simulink model "Last_version_po_STO"  (R2018a)
settings: Solver=FixedStepAuto  StartTime=0.0  StopTime=inf  FixedStep=1e-3  MaxStep=1e-4  RelTol=1e-3
undefined symbols (not defined in the file): D11, Delta
libraries: powerlib x118, simulink_extras x25, powerlib_meascontrol x18, simulink x8, xpcutilitieslib x2, xpcrtudplib x2, opclib x1, sldrtlib x1
(part 2 of 3)

== system Last_version_po_STO/fourier_filter20 ==
  In1 : Inport
  Complex to Real-Imag1 : ComplexToRealImag
  Degrees to Radians : simulink_extras/Transformations/Degrees to Radians
  Fourier1 : powerlib_meascontrol/Measurements/Fourier  Freq=50  n=1  InInit=[0, 0]  Ts=0
      settings: SourceProductName=Simscape Electrical
  Gain1 : Gain  Gain=1/sqrt(2)
  Magnitude-Angle to Complex1 : MagnitudeAngleToComplex
  RMS : Outport
  Real : Outport  Port=2
  Imag : Outport  Port=3
  Complex : Outport  Port=4
  Phase : Outport  Port=5
  wires:
  Fourier1/2 -> Degrees to Radians/1
  In1/1 -> Fourier1/1
  Magnitude-Angle to Complex1/1 -> Complex/1, Complex to Real-Imag1/1
  Complex to Real-Imag1/2 -> Imag/1
  Complex to Real-Imag1/1 -> Real/1
  Degrees to Radians/1 -> Phase/1, Magnitude-Angle to Complex1/2
  Fourier1/1 -> Gain1/1
  Gain1/1 -> RMS/1, Magnitude-Angle to Complex1/1

== system Last_version_po_STO/fourier_filter21 ==
  In1 : Inport
  Complex to Real-Imag1 : ComplexToRealImag
  Degrees to Radians : simulink_extras/Transformations/Degrees to Radians
  Fourier1 : powerlib_meascontrol/Measurements/Fourier  Freq=50  n=1  InInit=[0, 0]  Ts=0
      settings: SourceProductName=Simscape Electrical
  Gain1 : Gain  Gain=1/sqrt(2)
  Magnitude-Angle to Complex1 : MagnitudeAngleToComplex
  RMS : Outport
  Real : Outport  Port=2
  Imag : Outport  Port=3
  Complex : Outport  Port=4
  Phase : Outport  Port=5
  wires:
  Gain1/1 -> Magnitude-Angle to Complex1/1, RMS/1
  Fourier1/1 -> Gain1/1
  Degrees to Radians/1 -> Magnitude-Angle to Complex1/2, Phase/1
  Complex to Real-Imag1/1 -> Real/1
  Complex to Real-Imag1/2 -> Imag/1
  Magnitude-Angle to Complex1/1 -> Complex to Real-Imag1/1, Complex/1
  In1/1 -> Fourier1/1
  Fourier1/2 -> Degrees to Radians/1

== system Last_version_po_STO/fourier_filter22 ==
  In1 : Inport
  Complex to Real-Imag1 : ComplexToRealImag
  Degrees to Radians : simulink_extras/Transformations/Degrees to Radians
  Fourier1 : powerlib_meascontrol/Measurements/Fourier  Freq=50  n=1  InInit=[0, 0]  Ts=0
      settings: SourceProductName=Simscape Electrical
  Gain1 : Gain  Gain=1/sqrt(2)
  Magnitude-Angle to Complex1 : MagnitudeAngleToComplex
  RMS : Outport
  Real : Outport  Port=2
  Imag : Outport  Port=3
  Complex : Outport  Port=4
  Phase : Outport  Port=5
  wires:
  Fourier1/2 -> Degrees to Radians/1
  In1/1 -> Fourier1/1
  Magnitude-Angle to Complex1/1 -> Complex/1, Complex to Real-Imag1/1
  Complex to Real-Imag1/2 -> Imag/1
  Complex to Real-Imag1/1 -> Real/1
  Degrees to Radians/1 -> Phase/1, Magnitude-Angle to Complex1/2
  Fourier1/1 -> Gain1/1
  Gain1/1 -> RMS/1, Magnitude-Angle to Complex1/1

== system Last_version_po_STO/fourier_filter3 ==
  In1 : Inport
  Complex to Real-Imag1 : ComplexToRealImag
  Degrees to Radians : simulink_extras/Transformations/Degrees to Radians
  Fourier1 : powerlib_meascontrol/Measurements/Fourier  Freq=50  n=1  InInit=[0, 0]  Ts=0
      settings: SourceProductName=Simscape Electrical
  Gain1 : Gain  Gain=1/sqrt(2)
  Magnitude-Angle to Complex1 : MagnitudeAngleToComplex
  RMS : Outport
  Real : Outport  Port=2
  Imag : Outport  Port=3
  Complex : Outport  Port=4
  Phase : Outport  Port=5
  wires:
  Fourier1/2 -> Degrees to Radians/1
  In1/1 -> Fourier1/1
  Magnitude-Angle to Complex1/1 -> Complex/1, Complex to Real-Imag1/1
  Complex to Real-Imag1/2 -> Imag/1
  Complex to Real-Imag1/1 -> Real/1
  Degrees to Radians/1 -> Phase/1, Magnitude-Angle to Complex1/2
  Fourier1/1 -> Gain1/1
  Gain1/1 -> RMS/1, Magnitude-Angle to Complex1/1

== system Last_version_po_STO/fourier_filter4 ==
  In1 : Inport
  Complex to Real-Imag1 : ComplexToRealImag
  Degrees to Radians : simulink_extras/Transformations/Degrees to Radians
  Fourier1 : powerlib_meascontrol/Measurements/Fourier  Freq=50  n=1  InInit=[0, 0]  Ts=0
      settings: SourceProductName=Simscape Electrical
  Gain1 : Gain  Gain=1/sqrt(2)
  Magnitude-Angle to Complex1 : MagnitudeAngleToComplex
  RMS : Outport
  Real : Outport  Port=2
  Imag : Outport  Port=3
  Complex : Outport  Port=4
  Phase : Outport  Port=5
  wires:
  Fourier1/2 -> Degrees to Radians/1
  In1/1 -> Fourier1/1
  Magnitude-Angle to Complex1/1 -> Complex/1, Complex to Real-Imag1/1
  Complex to Real-Imag1/2 -> Imag/1
  Complex to Real-Imag1/1 -> Real/1
  Degrees to Radians/1 -> Phase/1, Magnitude-Angle to Complex1/2
  Fourier1/1 -> Gain1/1
  Gain1/1 -> RMS/1, Magnitude-Angle to Complex1/1

== system Last_version_po_STO/fourier_filter5 ==
  In1 : Inport
  Complex to Real-Imag1 : ComplexToRealImag
  Degrees to Radians : simulink_extras/Transformations/Degrees to Radians
  Fourier1 : powerlib_meascontrol/Measurements/Fourier  Freq=50  n=1  InInit=[0, 0]  Ts=0
      settings: SourceProductName=Simscape Electrical
  Gain1 : Gain  Gain=1/sqrt(2)
  Magnitude-Angle to Complex1 : MagnitudeAngleToComplex
  RMS : Outport
  Real : Outport  Port=2
  Imag : Outport  Port=3
  Complex : Outport  Port=4
  Phase : Outport  Port=5
  wires:
  Fourier1/2 -> Degrees to Radians/1
  In1/1 -> Fourier1/1
  Magnitude-Angle to Complex1/1 -> Complex/1, Complex to Real-Imag1/1
  Complex to Real-Imag1/2 -> Imag/1
  Complex to Real-Imag1/1 -> Real/1
  Degrees to Radians/1 -> Phase/1, Magnitude-Angle to Complex1/2
  Fourier1/1 -> Gain1/1
  Gain1/1 -> RMS/1, Magnitude-Angle to Complex1/1

== system Last_version_po_STO/fourier_filter6 ==
  In1 : Inport
  Complex to Real-Imag1 : ComplexToRealImag
  Degrees to Radians : simulink_extras/Transformations/Degrees to Radians
  Fourier1 : powerlib_meascontrol/Measurements/Fourier  Freq=50  n=1  InInit=[0, 0]  Ts=0
      settings: SourceProductName=Simscape Electrical
  Gain1 : Gain  Gain=1/sqrt(2)
  Magnitude-Angle to Complex1 : MagnitudeAngleToComplex
  RMS : Outport
  Real : Outport  Port=2
  Imag : Outport  Port=3
  Complex : Outport  Port=4
  Phase : Outport  Port=5
  wires:
  Fourier1/2 -> Degrees to Radians/1
  In1/1 -> Fourier1/1
  Magnitude-Angle to Complex1/1 -> Complex/1, Complex to Real-Imag1/1
  Complex to Real-Imag1/2 -> Imag/1
  Complex to Real-Imag1/1 -> Real/1
  Degrees to Radians/1 -> Phase/1, Magnitude-Angle to Complex1/2
  Fourier1/1 -> Gain1/1
  Gain1/1 -> RMS/1, Magnitude-Angle to Complex1/1

== system Last_version_po_STO/fourier_filter8 ==
  In1 : Inport
  Complex to Real-Imag1 : ComplexToRealImag
  Degrees to Radians : simulink_extras/Transformations/Degrees to Radians
  Fourier1 : powerlib_meascontrol/Measurements/Fourier  Freq=50  n=1  InInit=[0, 0]  Ts=0
      settings: SourceProductName=Simscape Electrical
  Gain1 : Gain  Gain=1/sqrt(2)
  Magnitude-Angle to Complex1 : MagnitudeAngleToComplex
  RMS : Outport
  Real : Outport  Port=2
  Imag : Outport  Port=3
  Complex : Outport  Port=4
  Phase : Outport  Port=5
  wires:
  Gain1/1 -> Magnitude-Angle to Complex1/1, RMS/1
  Fourier1/1 -> Gain1/1
  Degrees to Radians/1 -> Magnitude-Angle to Complex1/2, Phase/1
  Complex to Real-Imag1/1 -> Real/1
  Complex to Real-Imag1/2 -> Imag/1
  Magnitude-Angle to Complex1/1 -> Complex to Real-Imag1/1, Complex/1
  In1/1 -> Fourier1/1
  Fourier1/2 -> Degrees to Radians/1

== system Last_version_po_STO/relay_t ==
  In : Inport
  t_vv : Inport  Port=2
  Data Type Conversion : DataTypeConversion  OutDataTypeStr=double
  Integrator1 : Integrator  ExternalReset=rising  LimitOutput=on  UpperSaturationLimit=10000
  Logical Operator2 : Logic  Operator=NOT  AllPortsSameDT=off  OutDataTypeStr=boolean
  Relational Operator : RelationalOperator  Operator=>  OutDataTypeStr=boolean  RndMeth=Nearest
  Out : Outport
  wires:
  Logical Operator2/1 -> Integrator1/2
  In/1 -> Data Type Conversion/1, Logical Operator2/1
  Relational Operator/1 -> Out/1
  Integrator1/1 -> Relational Operator/1
  t_vv/1 -> Relational Operator/2
  Data Type Conversion/1 -> Integrator1/1

== system Last_version_po_STO/KZ_simulation/relay_t ==
  In : Inport
  t_vv : Inport  Port=2
  Data Type Conversion : DataTypeConversion  OutDataTypeStr=double
  Integrator1 : Integrator  ExternalReset=rising  LimitOutput=on  UpperSaturationLimit=10000
  Logical Operator2 : Logic  Operator=NOT  AllPortsSameDT=off  OutDataTypeStr=boolean
  Relational Operator : RelationalOperator  Operator=>  OutDataTypeStr=boolean  RndMeth=Nearest
  Out : Outport
  wires:
  Logical Operator2/1 -> Integrator1/2
  In/1 -> Data Type Conversion/1, Logical Operator2/1
  Relational Operator/1 -> Out/1
  Integrator1/1 -> Relational Operator/1
  t_vv/1 -> Relational Operator/2
  Data Type Conversion/1 -> Integrator1/1

== system Last_version_po_STO/KZ_simulation/relay_t1 ==
  In : Inport
  t_vv : Inport  Port=2
  Data Type Conversion : DataTypeConversion  OutDataTypeStr=double
  Integrator1 : Integrator  ExternalReset=rising  LimitOutput=on  UpperSaturationLimit=10000
  Logical Operator2 : Logic  Operator=NOT  AllPortsSameDT=off  OutDataTypeStr=boolean
  Relational Operator : RelationalOperator  Operator=>  OutDataTypeStr=boolean  RndMeth=Nearest
  Out : Outport
  wires:
  Data Type Conversion/1 -> Integrator1/1
  t_vv/1 -> Relational Operator/2
  Integrator1/1 -> Relational Operator/1
  Relational Operator/1 -> Out/1
  In/1 -> Logical Operator2/1, Data Type Conversion/1
  Logical Operator2/1 -> Integrator1/2

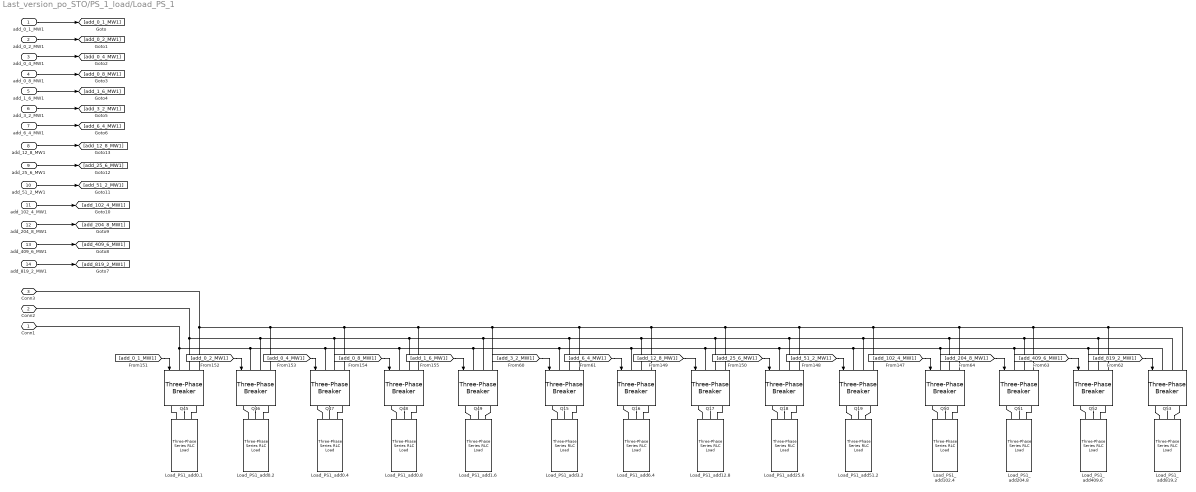
== system Last_version_po_STO/PS_1_load/Load_PS_1 ==
  add_0_1_MW1 : Inport
  add_0_2_MW1 : Inport  Port=2
  add_0_4_MW1 : Inport  Port=3
  add_0_8_MW1 : Inport  Port=4
  add_1_6_MW1 : Inport  Port=5
  add_3_2_MW1 : Inport  Port=6
  add_6_4_MW1 : Inport  Port=7
  add_12_8_MW1 : Inport  Port=8
  add_25_6_MW1 : Inport  Port=9
  add_51_2_MW1 : Inport  Port=10
  add_102_4_MW1 : Inport  Port=11
  add_204_8_MW1 : Inport  Port=12
  add_409_6_MW1 : Inport  Port=13
  add_819_2_MW1 : Inport  Port=14
  Load_PS1_add0.1 : powerlib/Elements/Three-Phase Series RLC Load  LConnTagsString=A|B|C  Configuration=Y (grounded)  NominalVoltage=330e3  Vabc=[1e3 1e3 1e3]  Vabcp=[1e3 1e3 1e3]  NominalFrequency=50  UnbalancedPower=off  ActivePower=0.1e6  InductivePower=0  CapacitivePower=0  Pabc=[10e3 9e3 11e3]  QLabc=[100 90 110]  QCabc=[100 90 110]  Pabcp=[10e3 9e3 11e3]  QLabcp=[100 90 110]  QCabcp=[100 90 110]  Measurements=None  LoadType=constant Z
      settings: SourceProductName=Simscape Electrical
  Load_PS1_add0.2 : powerlib/Elements/Three-Phase Series RLC Load  LConnTagsString=A|B|C  Configuration=Y (grounded)  NominalVoltage=330e3  Vabc=[1e3 1e3 1e3]  Vabcp=[1e3 1e3 1e3]  NominalFrequency=50  UnbalancedPower=off  ActivePower=0.2e6  InductivePower=0  CapacitivePower=0  Pabc=[10e3 9e3 11e3]  QLabc=[100 90 110]  QCabc=[100 90 110]  Pabcp=[10e3 9e3 11e3]  QLabcp=[100 90 110]  QCabcp=[100 90 110]  Measurements=None  LoadType=constant Z
      settings: SourceProductName=Simscape Electrical
  Load_PS1_add0.4 : powerlib/Elements/Three-Phase Series RLC Load  LConnTagsString=A|B|C  Configuration=Y (grounded)  NominalVoltage=330e3  Vabc=[1e3 1e3 1e3]  Vabcp=[1e3 1e3 1e3]  NominalFrequency=50  UnbalancedPower=off  ActivePower=0.4e6  InductivePower=0  CapacitivePower=0  Pabc=[10e3 9e3 11e3]  QLabc=[100 90 110]  QCabc=[100 90 110]  Pabcp=[10e3 9e3 11e3]  QLabcp=[100 90 110]  QCabcp=[100 90 110]  Measurements=None  LoadType=constant Z
      settings: SourceProductName=Simscape Electrical
  Load_PS1_add0.8 : powerlib/Elements/Three-Phase Series RLC Load  LConnTagsString=A|B|C  Configuration=Y (grounded)  NominalVoltage=330e3  Vabc=[1e3 1e3 1e3]  Vabcp=[1e3 1e3 1e3]  NominalFrequency=50  UnbalancedPower=off  ActivePower=0.8e6  InductivePower=0  CapacitivePower=0  Pabc=[10e3 9e3 11e3]  QLabc=[100 90 110]  QCabc=[100 90 110]  Pabcp=[10e3 9e3 11e3]  QLabcp=[100 90 110]  QCabcp=[100 90 110]  Measurements=None  LoadType=constant Z
      settings: SourceProductName=Simscape Electrical
  Load_PS1_add1.6 : powerlib/Elements/Three-Phase Series RLC Load  LConnTagsString=A|B|C  Configuration=Y (grounded)  NominalVoltage=330e3  Vabc=[1e3 1e3 1e3]  Vabcp=[1e3 1e3 1e3]  NominalFrequency=50  UnbalancedPower=off  ActivePower=1.6e6  InductivePower=0  CapacitivePower=0  Pabc=[10e3 9e3 11e3]  QLabc=[100 90 110]  QCabc=[100 90 110]  Pabcp=[10e3 9e3 11e3]  QLabcp=[100 90 110]  QCabcp=[100 90 110]  Measurements=None  LoadType=constant Z
      settings: SourceProductName=Simscape Electrical
  Load_PS1_add102.4 : powerlib/Elements/Three-Phase Series RLC Load  LConnTagsString=A|B|C  Configuration=Y (grounded)  NominalVoltage=330e3  Vabc=[1e3 1e3 1e3]  Vabcp=[1e3 1e3 1e3]  NominalFrequency=50  UnbalancedPower=off  ActivePower=102.4e6  InductivePower=0  CapacitivePower=0  Pabc=[10e3 9e3 11e3]  QLabc=[100 90 110]  QCabc=[100 90 110]  Pabcp=[10e3 9e3 11e3]  QLabcp=[100 90 110]  QCabcp=[100 90 110]  Measurements=None  LoadType=constant Z
      settings: SourceProductName=Simscape Electrical
  Load_PS1_add12.8 : powerlib/Elements/Three-Phase Series RLC Load  LConnTagsString=A|B|C  Configuration=Y (grounded)  NominalVoltage=330e3  Vabc=[1e3 1e3 1e3]  Vabcp=[1e3 1e3 1e3]  NominalFrequency=50  UnbalancedPower=off  ActivePower=12.8e6  InductivePower=0  CapacitivePower=0  Pabc=[10e3 9e3 11e3]  QLabc=[100 90 110]  QCabc=[100 90 110]  Pabcp=[10e3 9e3 11e3]  QLabcp=[100 90 110]  QCabcp=[100 90 110]  Measurements=None  LoadType=constant Z
      settings: SourceProductName=Simscape Electrical
  Load_PS1_add204.8 : powerlib/Elements/Three-Phase Series RLC Load  LConnTagsString=A|B|C  Configuration=Y (grounded)  NominalVoltage=330e3  Vabc=[1e3 1e3 1e3]  Vabcp=[1e3 1e3 1e3]  NominalFrequency=50  UnbalancedPower=off  ActivePower=204.8e6  InductivePower=0  CapacitivePower=0  Pabc=[10e3 9e3 11e3]  QLabc=[100 90 110]  QCabc=[100 90 110]  Pabcp=[10e3 9e3 11e3]  QLabcp=[100 90 110]  QCabcp=[100 90 110]  Measurements=None  LoadType=constant Z
      settings: SourceProductName=Simscape Electrical
  Load_PS1_add25.6 : powerlib/Elements/Three-Phase Series RLC Load  LConnTagsString=A|B|C  Configuration=Y (grounded)  NominalVoltage=330e3  Vabc=[1e3 1e3 1e3]  Vabcp=[1e3 1e3 1e3]  NominalFrequency=50  UnbalancedPower=off  ActivePower=25.6e6  InductivePower=0  CapacitivePower=0  Pabc=[10e3 9e3 11e3]  QLabc=[100 90 110]  QCabc=[100 90 110]  Pabcp=[10e3 9e3 11e3]  QLabcp=[100 90 110]  QCabcp=[100 90 110]  Measurements=None  LoadType=constant Z
      settings: SourceProductName=Simscape Electrical
  Load_PS1_add3.2 : powerlib/Elements/Three-Phase Series RLC Load  LConnTagsString=A|B|C  Configuration=Y (grounded)  NominalVoltage=330e3  Vabc=[1e3 1e3 1e3]  Vabcp=[1e3 1e3 1e3]  NominalFrequency=50  UnbalancedPower=off  ActivePower=3.2e6  InductivePower=0  CapacitivePower=0  Pabc=[10e3 9e3 11e3]  QLabc=[100 90 110]  QCabc=[100 90 110]  Pabcp=[10e3 9e3 11e3]  QLabcp=[100 90 110]  QCabcp=[100 90 110]  Measurements=None  LoadType=constant Z
      settings: SourceProductName=Simscape Electrical
  Load_PS1_add409.6 : powerlib/Elements/Three-Phase Series RLC Load  LConnTagsString=A|B|C  Configuration=Y (grounded)  NominalVoltage=330e3  Vabc=[1e3 1e3 1e3]  Vabcp=[1e3 1e3 1e3]  NominalFrequency=50  UnbalancedPower=off  ActivePower=409.6e6  InductivePower=0  CapacitivePower=0  Pabc=[10e3 9e3 11e3]  QLabc=[100 90 110]  QCabc=[100 90 110]  Pabcp=[10e3 9e3 11e3]  QLabcp=[100 90 110]  QCabcp=[100 90 110]  Measurements=None  LoadType=constant Z
      settings: SourceProductName=Simscape Electrical
  Load_PS1_add51.2 : powerlib/Elements/Three-Phase Series RLC Load  LConnTagsString=A|B|C  Configuration=Y (grounded)  NominalVoltage=330e3  Vabc=[1e3 1e3 1e3]  Vabcp=[1e3 1e3 1e3]  NominalFrequency=50  UnbalancedPower=off  ActivePower=51.2e6  InductivePower=0  CapacitivePower=0  Pabc=[10e3 9e3 11e3]  QLabc=[100 90 110]  QCabc=[100 90 110]  Pabcp=[10e3 9e3 11e3]  QLabcp=[100 90 110]  QCabcp=[100 90 110]  Measurements=None  LoadType=constant Z
      settings: SourceProductName=Simscape Electrical
  Load_PS1_add6.4 : powerlib/Elements/Three-Phase Series RLC Load  LConnTagsString=A|B|C  Configuration=Y (grounded)  NominalVoltage=330e3  Vabc=[1e3 1e3 1e3]  Vabcp=[1e3 1e3 1e3]  NominalFrequency=50  UnbalancedPower=off  ActivePower=6.4e6  InductivePower=0  CapacitivePower=0  Pabc=[10e3 9e3 11e3]  QLabc=[100 90 110]  QCabc=[100 90 110]  Pabcp=[10e3 9e3 11e3]  QLabcp=[100 90 110]  QCabcp=[100 90 110]  Measurements=None  LoadType=constant Z
      settings: SourceProductName=Simscape Electrical
  Load_PS1_add819.2 : powerlib/Elements/Three-Phase Series RLC Load  LConnTagsString=A|B|C  Configuration=Y (grounded)  NominalVoltage=330e3  Vabc=[1e3 1e3 1e3]  Vabcp=[1e3 1e3 1e3]  NominalFrequency=50  UnbalancedPower=off  ActivePower=819.2e6  InductivePower=0  CapacitivePower=0  Pabc=[10e3 9e3 11e3]  QLabc=[100 90 110]  QCabc=[100 90 110]  Pabcp=[10e3 9e3 11e3]  QLabcp=[100 90 110]  QCabcp=[100 90 110]  Measurements=None  LoadType=constant Z
      settings: SourceProductName=Simscape Electrical
  Q{15..19,45..53} (14 alike) : powerlib/Elements/Three-Phase Breaker  InitialState=open  SwitchA=on  SwitchB=on  SwitchC=on  SwitchTimes="[1/60  5/60]"  External=on  BreakerResistance=0.01  SnubberResistance=1e6  SnubberCapacitance=inf  Measurements=None
      settings: SourceProductName=Simscape Electrical
  Conn1 : PMIOPort  Side=Left
  Conn2 : PMIOPort  Port=2  Side=Left
  Conn3 : PMIOPort  Port=3  Side=Left
  wires:
  [add_0_8_MW1] -> Q48/1
  [add_1_6_MW1] -> Q49/1
  [add_6_4_MW1] -> Q16/1
  [add_3_2_MW1] -> Q15/1
  [add_204_8_MW1] -> Q51/1
  [add_25_6_MW1] -> Q18/1
  [add_0_4_MW1] -> Q47/1
  [add_0_1_MW1] -> Q45/1
  [add_0_2_MW1] -> Q46/1
  [add_409_6_MW1] -> Q52/1
  [add_51_2_MW1] -> Q19/1
  [add_819_2_MW1] -> Q53/1
  [add_12_8_MW1] -> Q17/1
  [add_102_4_MW1] -> Q50/1
  add_0_1_MW1/1 -> [add_0_1_MW1]
  add_0_2_MW1/1 -> [add_0_2_MW1]
  add_0_4_MW1/1 -> [add_0_4_MW1]
  add_0_8_MW1/1 -> [add_0_8_MW1]
  add_1_6_MW1/1 -> [add_1_6_MW1]
  add_3_2_MW1/1 -> [add_3_2_MW1]
  add_6_4_MW1/1 -> [add_6_4_MW1]
  add_25_6_MW1/1 -> [add_25_6_MW1]
  add_51_2_MW1/1 -> [add_51_2_MW1]
  add_102_4_MW1/1 -> [add_102_4_MW1]
  add_204_8_MW1/1 -> [add_204_8_MW1]
  add_409_6_MW1/1 -> [add_409_6_MW1]
  add_819_2_MW1/1 -> [add_819_2_MW1]
  add_12_8_MW1/1 -> [add_12_8_MW1]
  connections:
  Q52/LConn1 -- Q48/LConn1 -- Q47/LConn1 -- Q46/LConn1 -- Conn1/RConn1 -- Q45/LConn1 -- Q49/LConn1 -- Q15/LConn1 -- Q16/LConn1 -- Q17/LConn1 -- Q18/LConn1 -- Q19/LConn1 -- Q50/LConn1 -- Q51/LConn1 -- Q53/LConn1
  Load_PS1_add12.8/LConn2 -- Q17/RConn2
  Q52/LConn3 -- Q48/LConn3 -- Q47/LConn3 -- Q46/LConn3 -- Conn3/RConn1 -- Q45/LConn3 -- Q49/LConn3 -- Q15/LConn3 -- Q16/LConn3 -- Q17/LConn3 -- Q18/LConn3 -- Q19/LConn3 -- Q50/LConn3 -- Q51/LConn3 -- Q53/LConn3
  Q52/LConn2 -- Q48/LConn2 -- Q47/LConn2 -- Q46/LConn2 -- Conn2/RConn1 -- Q45/LConn2 -- Q49/LConn2 -- Q15/LConn2 -- Q16/LConn2 -- Q17/LConn2 -- Q18/LConn2 -- Q19/LConn2 -- Q50/LConn2 -- Q51/LConn2 -- Q53/LConn2
  Q49/RConn1 -- Load_PS1_add1.6/LConn1
  Load_PS1_add6.4/LConn1 -- Q16/RConn1
  Q53/RConn1 -- Load_PS1_add819.2/LConn1
  Load_PS1_add1.6/LConn2 -- Q49/RConn2
  Load_PS1_add409.6/LConn3 -- Q52/RConn3
  Load_PS1_add0.2/LConn1 -- Q46/RConn1
  Load_PS1_add102.4/LConn3 -- Q50/RConn3
  Q45/RConn2 -- Load_PS1_add0.1/LConn2
  Load_PS1_add0.1/LConn3 -- Q45/RConn3
  Load_PS1_add0.4/LConn1 -- Q47/RConn1
  Q48/RConn2 -- Load_PS1_add0.8/LConn2
  Q49/RConn3 -- Load_PS1_add1.6/LConn3
  Load_PS1_add0.8/LConn3 -- Q48/RConn3
  Q16/RConn2 -- Load_PS1_add6.4/LConn2
  Q19/RConn3 -- Load_PS1_add51.2/LConn3
  Load_PS1_add0.8/LConn1 -- Q48/RConn1
  Q53/RConn3 -- Load_PS1_add819.2/LConn3
  Q19/RConn1 -- Load_PS1_add51.2/LConn1
  Load_PS1_add25.6/LConn1 -- Q18/RConn1
  Load_PS1_add25.6/LConn3 -- Q18/RConn3
  Load_PS1_add0.4/LConn2 -- Q47/RConn2
  Load_PS1_add12.8/LConn1 -- Q17/RConn1
  Load_PS1_add102.4/LConn1 -- Q50/RConn1
  Load_PS1_add819.2/LConn2 -- Q53/RConn2
  Load_PS1_add0.1/LConn1 -- Q45/RConn1
  Q52/RConn2 -- Load_PS1_add409.6/LConn2
  Q18/RConn2 -- Load_PS1_add25.6/LConn2
  Load_PS1_add0.4/LConn3 -- Q47/RConn3
  Load_PS1_add6.4/LConn3 -- Q16/RConn3
  Q46/RConn2 -- Load_PS1_add0.2/LConn2
  Load_PS1_add409.6/LConn1 -- Q52/RConn1
  Load_PS1_add51.2/LConn2 -- Q19/RConn2
  Load_PS1_add3.2/LConn3 -- Q15/RConn3
  Load_PS1_add0.2/LConn3 -- Q46/RConn3
  Load_PS1_add204.8/LConn3 -- Q51/RConn3
  Load_PS1_add3.2/LConn1 -- Q15/RConn1
  Load_PS1_add204.8/LConn2 -- Q51/RConn2
  Load_PS1_add12.8/LConn3 -- Q17/RConn3
  Q50/RConn2 -- Load_PS1_add102.4/LConn2
  Load_PS1_add204.8/LConn1 -- Q51/RConn1
  Load_PS1_add3.2/LConn2 -- Q15/RConn2

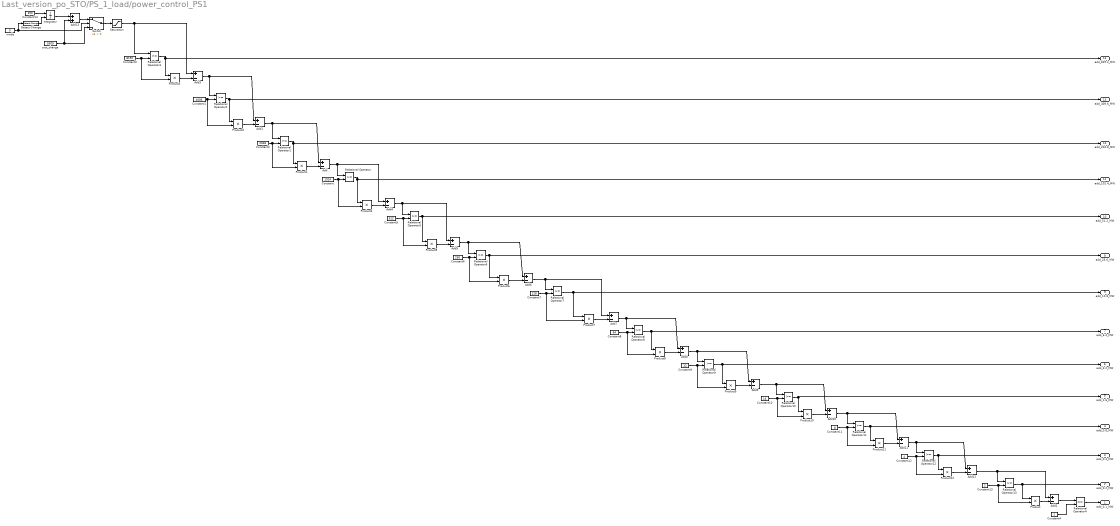
== system Last_version_po_STO/PS_1_load/power_control_PS1 ==
  Add{,1..12} (13 alike) : Sum  Inputs=+-
  Add13 : Sum
  Constant : Constant  Value=1024
  Constant1 : Constant  Value=4096
  Constant10 : Constant  Value=16
  Constant11 : Constant  Value=8
  Constant12 : Constant  Value=4
  Constant13 : Constant  Value=2
  Constant14 : Constant  Value=350
  Constant2 : Constant  Value=2048
  Constant3 : Constant  Value=8192
  Constant4 : Constant
  Constant5 : Constant  Value=512
  Constant6 : Constant  Value=256
  Constant7 : Constant  Value=128
  Constant8 : Constant  Value=64
  Constant9 : Constant  Value=32
  Detect Change : simulink/Logic and Bit Operations/Detect Change  vinit=0  OutDataTypeStr=boolean
  Integrator : Integrator  ExternalReset=rising
  Product{,1..12} (13 alike) : Product
  Relational Operator{,1..3,5..13} (13 alike) : RelationalOperator  OutDataTypeStr=boolean  RndMeth=Simplest
  Relational Operator4 : RelationalOperator  Operator===  OutDataTypeStr=boolean  RndMeth=Simplest
  Saturation : Saturate  UpperLimit=10000  LowerLimit=0
  Switch : Switch  Criteria=u2 > Threshold
  cnst_change : Constant  Value=5509
  mode : Constant  Value=0
  add_0.1_MW : Outport
  add_0.2_MW : Outport  Port=2
  add_0.4_MW : Outport  Port=3
  add_0.8_MW : Outport  Port=4
  add_1.6_MW : Outport  Port=5
  add_3.2_MW : Outport  Port=6
  add_6.4_MW : Outport  Port=7
  add_12.8_MW : Outport  Port=8
  add_25.6_MW : Outport  Port=9
  add_51.2_MW : Outport  Port=10
  add_102.4_MW : Outport  Port=11
  add_204.8_MW : Outport  Port=12
  add_409.6_MW : Outport  Port=13
  add_819.2_MW : Outport  Port=14
  wires:
  Constant3/1 -> Relational Operator3/2, Product3/2
  Add2/1 -> Relational Operator4/1
  Relational Operator2/1 -> Product2/1, add_409.6_MW/1
  Add1/1 -> Relational Operator1/1, Add/1
  Constant1/1 -> Relational Operator2/2, Product2/2
  Product2/1 -> Add1/2
  Relational Operator4/1 -> add_0.1_MW/1
  Constant4/1 -> Relational Operator4/2
  Product1/1 -> Add/2
  Product/1 -> Add2/2
  Add/1 -> Add4/1, Relational Operator/1
  Relational Operator/1 -> add_102.4_MW/1, Product4/1
  Constant2/1 -> Relational Operator1/2, Product1/2
  Relational Operator1/1 -> Product1/1, add_204.8_MW/1
  Constant/1 -> Product4/2, Relational Operator/2
  Product3/1 -> Add3/2
  Add3/1 -> Relational Operator2/1, Add1/1
  Relational Operator3/1 -> Product3/1, add_819.2_MW/1
  Constant5/1 -> Product5/2, Relational Operator5/2
  Add4/1 -> Add5/1, Relational Operator5/1
  Product4/1 -> Add4/2
  Product5/1 -> Add5/2
  Add5/1 -> Relational Operator6/1, Add6/1
  Constant6/1 -> Product6/2, Relational Operator6/2
  Constant7/1 -> Product7/2, Relational Operator7/2
  Add6/1 -> Add7/1, Relational Operator7/1
  Product6/1 -> Add6/2
  Relational Operator5/1 -> Product5/1, add_51.2_MW/1
  Relational Operator6/1 -> add_25.6_MW/1, Product6/1
  Product7/1 -> Add7/2
  Add7/1 -> Add8/1, Relational Operator8/1
  Constant8/1 -> Product8/2, Relational Operator8/2
  Constant9/1 -> Product9/2, Relational Operator9/2
  Add8/1 -> Add9/1, Relational Operator9/1
  Product8/1 -> Add8/2
  Product9/1 -> Add9/2
  Add9/1 -> Add10/1, Relational Operator10/1
  Constant10/1 -> Product10/2, Relational Operator10/2
  Constant11/1 -> Product11/2, Relational Operator11/2
  Add10/1 -> Add11/1, Relational Operator11/1
  Product10/1 -> Add10/2
  Product11/1 -> Add11/2
  Add11/1 -> Add12/1, Relational Operator12/1
  Constant12/1 -> Product12/2, Relational Operator12/2
  Constant13/1 -> Product/2, Relational Operator13/2
  Add12/1 -> Add2/1, Relational Operator13/1
  Product12/1 -> Add12/2
  Relational Operator7/1 -> add_12.8_MW/1, Product7/1
  Relational Operator8/1 -> add_6.4_MW/1, Product8/1
  Relational Operator9/1 -> add_3.2_MW/1, Product9/1
  Relational Operator10/1 -> add_1.6_MW/1, Product10/1
  Relational Operator11/1 -> add_0.8_MW/1, Product11/1
  Relational Operator12/1 -> add_0.4_MW/1, Product12/1
  Relational Operator13/1 -> add_0.2_MW/1, Product/1
  Constant14/1 -> Integrator/1
  cnst_change/1 -> Switch/3, Add13/2
  Saturation/1 -> Relational Operator3/1, Add3/1
  Switch/1 -> Saturation/1
  Add13/1 -> Switch/1
  Integrator/1 -> Add13/1
  mode/1 -> Detect Change/1, Switch/2
  Detect Change/1 -> Integrator/2

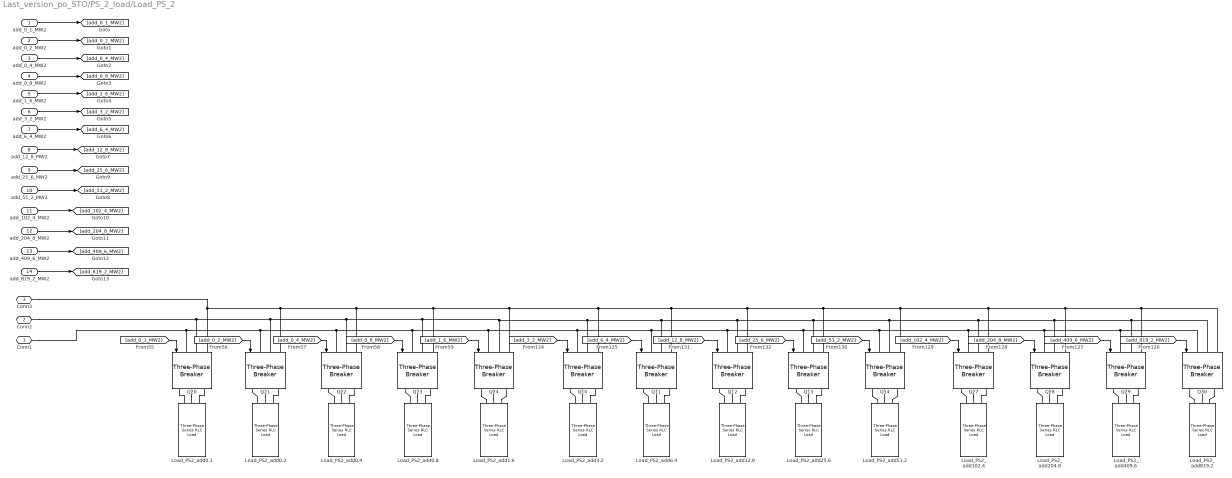
== system Last_version_po_STO/PS_2_load/Load_PS_2 ==
  add_0_1_MW2 : Inport
  add_0_2_MW2 : Inport  Port=2
  add_0_4_MW2 : Inport  Port=3
  add_0_8_MW2 : Inport  Port=4
  add_1_6_MW2 : Inport  Port=5
  add_3_2_MW2 : Inport  Port=6
  add_6_4_MW2 : Inport  Port=7
  add_12_8_MW2 : Inport  Port=8
  add_25_6_MW2 : Inport  Port=9
  add_51_2_MW2 : Inport  Port=10
  add_102_4_MW2 : Inport  Port=11
  add_204_8_MW2 : Inport  Port=12
  add_409_6_MW2 : Inport  Port=13
  add_819_2_MW2 : Inport  Port=14
  Load_PS2_add0.1 : powerlib/Elements/Three-Phase Series RLC Load  LConnTagsString=A|B|C  Configuration=Y (grounded)  NominalVoltage=330e3  Vabc=[1e3 1e3 1e3]  Vabcp=[1e3 1e3 1e3]  NominalFrequency=50  UnbalancedPower=off  ActivePower=0.1e6  InductivePower=0  CapacitivePower=0  Pabc=[10e3 9e3 11e3]  QLabc=[100 90 110]  QCabc=[100 90 110]  Pabcp=[10e3 9e3 11e3]  QLabcp=[100 90 110]  QCabcp=[100 90 110]  Measurements=None  LoadType=constant Z
      settings: SourceProductName=Simscape Electrical
  Load_PS2_add0.2 : powerlib/Elements/Three-Phase Series RLC Load  LConnTagsString=A|B|C  Configuration=Y (grounded)  NominalVoltage=330e3  Vabc=[1e3 1e3 1e3]  Vabcp=[1e3 1e3 1e3]  NominalFrequency=50  UnbalancedPower=off  ActivePower=0.2e6  InductivePower=0  CapacitivePower=0  Pabc=[10e3 9e3 11e3]  QLabc=[100 90 110]  QCabc=[100 90 110]  Pabcp=[10e3 9e3 11e3]  QLabcp=[100 90 110]  QCabcp=[100 90 110]  Measurements=None  LoadType=constant Z
      settings: SourceProductName=Simscape Electrical
  Load_PS2_add0.4 : powerlib/Elements/Three-Phase Series RLC Load  LConnTagsString=A|B|C  Configuration=Y (grounded)  NominalVoltage=330e3  Vabc=[1e3 1e3 1e3]  Vabcp=[1e3 1e3 1e3]  NominalFrequency=50  UnbalancedPower=off  ActivePower=0.4e6  InductivePower=0  CapacitivePower=0  Pabc=[10e3 9e3 11e3]  QLabc=[100 90 110]  QCabc=[100 90 110]  Pabcp=[10e3 9e3 11e3]  QLabcp=[100 90 110]  QCabcp=[100 90 110]  Measurements=None  LoadType=constant Z
      settings: SourceProductName=Simscape Electrical
  Load_PS2_add0.8 : powerlib/Elements/Three-Phase Series RLC Load  LConnTagsString=A|B|C  Configuration=Y (grounded)  NominalVoltage=330e3  Vabc=[1e3 1e3 1e3]  Vabcp=[1e3 1e3 1e3]  NominalFrequency=50  UnbalancedPower=off  ActivePower=0.8e6  InductivePower=0  CapacitivePower=0  Pabc=[10e3 9e3 11e3]  QLabc=[100 90 110]  QCabc=[100 90 110]  Pabcp=[10e3 9e3 11e3]  QLabcp=[100 90 110]  QCabcp=[100 90 110]  Measurements=None  LoadType=constant Z
      settings: SourceProductName=Simscape Electrical
  Load_PS2_add1.6 : powerlib/Elements/Three-Phase Series RLC Load  LConnTagsString=A|B|C  Configuration=Y (grounded)  NominalVoltage=330e3  Vabc=[1e3 1e3 1e3]  Vabcp=[1e3 1e3 1e3]  NominalFrequency=50  UnbalancedPower=off  ActivePower=1.6e6  InductivePower=0  CapacitivePower=0  Pabc=[10e3 9e3 11e3]  QLabc=[100 90 110]  QCabc=[100 90 110]  Pabcp=[10e3 9e3 11e3]  QLabcp=[100 90 110]  QCabcp=[100 90 110]  Measurements=None  LoadType=constant Z
      settings: SourceProductName=Simscape Electrical
  Load_PS2_add102.4 : powerlib/Elements/Three-Phase Series RLC Load  LConnTagsString=A|B|C  Configuration=Y (grounded)  NominalVoltage=330e3  Vabc=[1e3 1e3 1e3]  Vabcp=[1e3 1e3 1e3]  NominalFrequency=50  UnbalancedPower=off  ActivePower=102.4e6  InductivePower=0  CapacitivePower=0  Pabc=[10e3 9e3 11e3]  QLabc=[100 90 110]  QCabc=[100 90 110]  Pabcp=[10e3 9e3 11e3]  QLabcp=[100 90 110]  QCabcp=[100 90 110]  Measurements=None  LoadType=constant Z
      settings: SourceProductName=Simscape Electrical
  Load_PS2_add12.8 : powerlib/Elements/Three-Phase Series RLC Load  LConnTagsString=A|B|C  Configuration=Y (grounded)  NominalVoltage=330e3  Vabc=[1e3 1e3 1e3]  Vabcp=[1e3 1e3 1e3]  NominalFrequency=50  UnbalancedPower=off  ActivePower=12.8e6  InductivePower=0  CapacitivePower=0  Pabc=[10e3 9e3 11e3]  QLabc=[100 90 110]  QCabc=[100 90 110]  Pabcp=[10e3 9e3 11e3]  QLabcp=[100 90 110]  QCabcp=[100 90 110]  Measurements=None  LoadType=constant Z
      settings: SourceProductName=Simscape Electrical
  Load_PS2_add204.8 : powerlib/Elements/Three-Phase Series RLC Load  LConnTagsString=A|B|C  Configuration=Y (grounded)  NominalVoltage=330e3  Vabc=[1e3 1e3 1e3]  Vabcp=[1e3 1e3 1e3]  NominalFrequency=50  UnbalancedPower=off  ActivePower=204.8e6  InductivePower=0  CapacitivePower=0  Pabc=[10e3 9e3 11e3]  QLabc=[100 90 110]  QCabc=[100 90 110]  Pabcp=[10e3 9e3 11e3]  QLabcp=[100 90 110]  QCabcp=[100 90 110]  Measurements=None  LoadType=constant Z
      settings: SourceProductName=Simscape Electrical
  Load_PS2_add25.6 : powerlib/Elements/Three-Phase Series RLC Load  LConnTagsString=A|B|C  Configuration=Y (grounded)  NominalVoltage=330e3  Vabc=[1e3 1e3 1e3]  Vabcp=[1e3 1e3 1e3]  NominalFrequency=50  UnbalancedPower=off  ActivePower=25.6e6  InductivePower=0  CapacitivePower=0  Pabc=[10e3 9e3 11e3]  QLabc=[100 90 110]  QCabc=[100 90 110]  Pabcp=[10e3 9e3 11e3]  QLabcp=[100 90 110]  QCabcp=[100 90 110]  Measurements=None  LoadType=constant Z
      settings: SourceProductName=Simscape Electrical
  Load_PS2_add3.2 : powerlib/Elements/Three-Phase Series RLC Load  LConnTagsString=A|B|C  Configuration=Y (grounded)  NominalVoltage=330e3  Vabc=[1e3 1e3 1e3]  Vabcp=[1e3 1e3 1e3]  NominalFrequency=50  UnbalancedPower=off  ActivePower=3.2e6  InductivePower=0  CapacitivePower=0  Pabc=[10e3 9e3 11e3]  QLabc=[100 90 110]  QCabc=[100 90 110]  Pabcp=[10e3 9e3 11e3]  QLabcp=[100 90 110]  QCabcp=[100 90 110]  Measurements=None  LoadType=constant Z
      settings: SourceProductName=Simscape Electrical
  Load_PS2_add409.6 : powerlib/Elements/Three-Phase Series RLC Load  LConnTagsString=A|B|C  Configuration=Y (grounded)  NominalVoltage=330e3  Vabc=[1e3 1e3 1e3]  Vabcp=[1e3 1e3 1e3]  NominalFrequency=50  UnbalancedPower=off  ActivePower=409.6e6  InductivePower=0  CapacitivePower=0  Pabc=[10e3 9e3 11e3]  QLabc=[100 90 110]  QCabc=[100 90 110]  Pabcp=[10e3 9e3 11e3]  QLabcp=[100 90 110]  QCabcp=[100 90 110]  Measurements=None  LoadType=constant Z
      settings: SourceProductName=Simscape Electrical
  Load_PS2_add51.2 : powerlib/Elements/Three-Phase Series RLC Load  LConnTagsString=A|B|C  Configuration=Y (grounded)  NominalVoltage=330e3  Vabc=[1e3 1e3 1e3]  Vabcp=[1e3 1e3 1e3]  NominalFrequency=50  UnbalancedPower=off  ActivePower=51.2e6  InductivePower=0  CapacitivePower=0  Pabc=[10e3 9e3 11e3]  QLabc=[100 90 110]  QCabc=[100 90 110]  Pabcp=[10e3 9e3 11e3]  QLabcp=[100 90 110]  QCabcp=[100 90 110]  Measurements=None  LoadType=constant Z
      settings: SourceProductName=Simscape Electrical
  Load_PS2_add6.4 : powerlib/Elements/Three-Phase Series RLC Load  LConnTagsString=A|B|C  Configuration=Y (grounded)  NominalVoltage=330e3  Vabc=[1e3 1e3 1e3]  Vabcp=[1e3 1e3 1e3]  NominalFrequency=50  UnbalancedPower=off  ActivePower=6.4e6  InductivePower=0  CapacitivePower=0  Pabc=[10e3 9e3 11e3]  QLabc=[100 90 110]  QCabc=[100 90 110]  Pabcp=[10e3 9e3 11e3]  QLabcp=[100 90 110]  QCabcp=[100 90 110]  Measurements=None  LoadType=constant Z
      settings: SourceProductName=Simscape Electrical
  Load_PS2_add819.2 : powerlib/Elements/Three-Phase Series RLC Load  LConnTagsString=A|B|C  Configuration=Y (grounded)  NominalVoltage=330e3  Vabc=[1e3 1e3 1e3]  Vabcp=[1e3 1e3 1e3]  NominalFrequency=50  UnbalancedPower=off  ActivePower=819.2e6  InductivePower=0  CapacitivePower=0  Pabc=[10e3 9e3 11e3]  QLabc=[100 90 110]  QCabc=[100 90 110]  Pabcp=[10e3 9e3 11e3]  QLabcp=[100 90 110]  QCabcp=[100 90 110]  Measurements=None  LoadType=constant Z
      settings: SourceProductName=Simscape Electrical
  Q{10..14,20..24,27..30} (14 alike) : powerlib/Elements/Three-Phase Breaker  InitialState=open  SwitchA=on  SwitchB=on  SwitchC=on  SwitchTimes="[1/60  5/60]"  External=on  BreakerResistance=0.01  SnubberResistance=1e6  SnubberCapacitance=inf  Measurements=None
      settings: SourceProductName=Simscape Electrical
  Conn1 : PMIOPort  Side=Left
  Conn2 : PMIOPort  Port=2  Side=Left
  Conn3 : PMIOPort  Port=3  Side=Left
  wires:
  [add_0_8_MW2] -> Q23/1
  [add_204_8_MW2] -> Q28/1
  [add_25_6_MW2] -> Q13/1
  [add_1_6_MW2] -> Q24/1
  [add_0_4_MW2] -> Q22/1
  [add_0_2_MW2] -> Q21/1
  [add_819_2_MW2] -> Q30/1
  [add_6_4_MW2] -> Q11/1
  [add_409_6_MW2] -> Q29/1
  [add_51_2_MW2] -> Q14/1
  [add_0_1_MW2] -> Q20/1
  [add_102_4_MW2] -> Q27/1
  [add_3_2_MW2] -> Q10/1
  [add_12_8_MW2] -> Q12/1
  add_0_1_MW2/1 -> [add_0_1_MW2]
  add_0_4_MW2/1 -> [add_0_4_MW2]
  add_0_2_MW2/1 -> [add_0_2_MW2]
  add_0_8_MW2/1 -> [add_0_8_MW2]
  add_1_6_MW2/1 -> [add_1_6_MW2]
  add_3_2_MW2/1 -> [add_3_2_MW2]
  add_6_4_MW2/1 -> [add_6_4_MW2]
  add_12_8_MW2/1 -> [add_12_8_MW2]
  add_25_6_MW2/1 -> [add_25_6_MW2]
  add_51_2_MW2/1 -> [add_51_2_MW2]
  add_102_4_MW2/1 -> [add_102_4_MW2]
  add_204_8_MW2/1 -> [add_204_8_MW2]
  add_409_6_MW2/1 -> [add_409_6_MW2]
  add_819_2_MW2/1 -> [add_819_2_MW2]
  connections:
  Load_PS2_add204.8/LConn2 -- Q28/RConn2
  Q11/RConn2 -- Load_PS2_add6.4/LConn2
  Q24/LConn3 -- Q29/LConn3 -- Q30/LConn3 -- Q28/LConn3 -- Q27/LConn3 -- Q14/LConn3 -- Q13/LConn3 -- Q12/LConn3 -- Q11/LConn3 -- Q10/LConn3 -- Q23/LConn3 -- Q22/LConn3 -- Q21/LConn3 -- Conn3/RConn1 -- Q20/LConn3
  Q24/LConn2 -- Q29/LConn2 -- Q30/LConn2 -- Q28/LConn2 -- Q27/LConn2 -- Q14/LConn2 -- Q13/LConn2 -- Q12/LConn2 -- Q11/LConn2 -- Q10/LConn2 -- Q23/LConn2 -- Q22/LConn2 -- Q21/LConn2 -- Conn2/RConn1 -- Q20/LConn2
  Load_PS2_add204.8/LConn3 -- Q28/RConn3
  Load_PS2_add0.1/LConn1 -- Q20/RConn1
  Q23/LConn1 -- Q29/LConn1 -- Q30/LConn1 -- Q28/LConn1 -- Q27/LConn1 -- Q14/LConn1 -- Q13/LConn1 -- Q12/LConn1 -- Q11/LConn1 -- Q10/LConn1 -- Q24/LConn1 -- Q22/LConn1 -- Q21/LConn1 -- Conn1/RConn1 -- Q20/LConn1
  Load_PS2_add25.6/LConn1 -- Q13/RConn1
  Load_PS2_add0.1/LConn3 -- Q20/RConn3
  Load_PS2_add0.8/LConn3 -- Q23/RConn3
  Q27/RConn2 -- Load_PS2_add102.4/LConn2
  Q30/RConn1 -- Load_PS2_add819.2/LConn1
  Load_PS2_add0.2/LConn3 -- Q21/RConn3
  Load_PS2_add1.6/LConn2 -- Q24/RConn2
  Q20/RConn2 -- Load_PS2_add0.1/LConn2
  Q24/RConn1 -- Load_PS2_add1.6/LConn1
  Load_PS2_add0.8/LConn1 -- Q23/RConn1
  Load_PS2_add0.4/LConn2 -- Q22/RConn2
  Q24/RConn3 -- Load_PS2_add1.6/LConn3
  Q29/RConn2 -- Load_PS2_add409.6/LConn2
  Q21/RConn2 -- Load_PS2_add0.2/LConn2
  Load_PS2_add3.2/LConn2 -- Q10/RConn2
  Q14/RConn1 -- Load_PS2_add51.2/LConn1
  Load_PS2_add25.6/LConn3 -- Q13/RConn3
  Load_PS2_add12.8/LConn3 -- Q12/RConn3
  Load_PS2_add12.8/LConn2 -- Q12/RConn2
  Load_PS2_add6.4/LConn3 -- Q11/RConn3
  Q14/RConn3 -- Load_PS2_add51.2/LConn3
  Q30/RConn3 -- Load_PS2_add819.2/LConn3
  Load_PS2_add102.4/LConn1 -- Q27/RConn1
  Load_PS2_add204.8/LConn1 -- Q28/RConn1
  Load_PS2_add6.4/LConn1 -- Q11/RConn1
  Load_PS2_add409.6/LConn3 -- Q29/RConn3
  Load_PS2_add0.2/LConn1 -- Q21/RConn1
  Q13/RConn2 -- Load_PS2_add25.6/LConn2
  Load_PS2_add12.8/LConn1 -- Q12/RConn1
  Load_PS2_add3.2/LConn3 -- Q10/RConn3
  Load_PS2_add819.2/LConn2 -- Q30/RConn2
  Load_PS2_add3.2/LConn1 -- Q10/RConn1
  Load_PS2_add409.6/LConn1 -- Q29/RConn1
  Q23/RConn2 -- Load_PS2_add0.8/LConn2
  Load_PS2_add102.4/LConn3 -- Q27/RConn3
  Load_PS2_add0.4/LConn3 -- Q22/RConn3
  Load_PS2_add0.4/LConn1 -- Q22/RConn1
  Load_PS2_add51.2/LConn2 -- Q14/RConn2

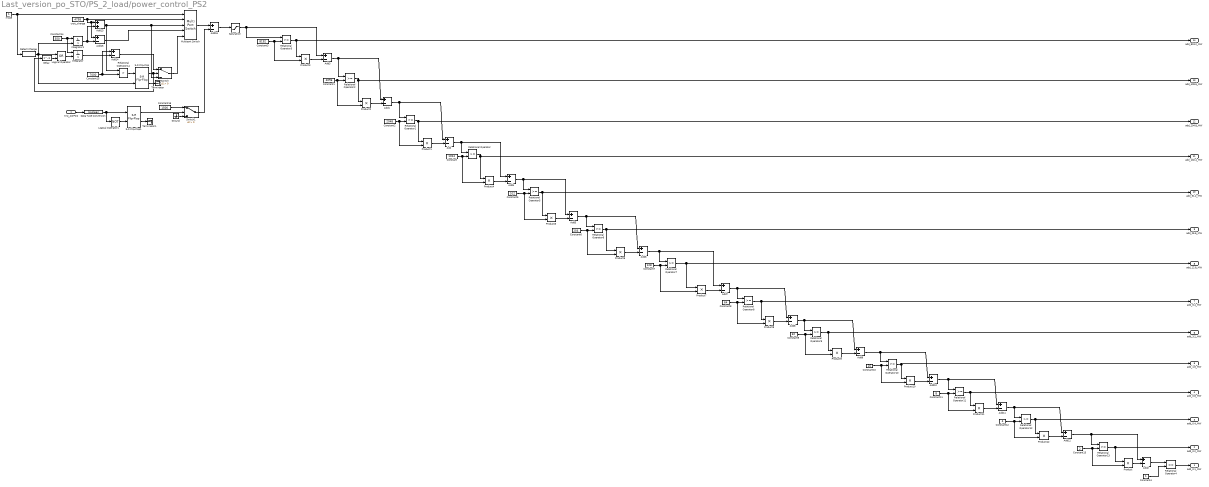
== system Last_version_po_STO/PS_2_load/power_control_PS2 ==
  trip_AOPO2 : Inport
  Add{,1..12,14..16} (16 alike) : Sum  Inputs=+-
  Add13 : Sum
  Constant : Constant  Value=1024
  Constant1 : Constant  Value=4096
  Constant10 : Constant  Value=16
  Constant11 : Constant  Value=8
  Constant12 : Constant  Value=4
  Constant13 : Constant  Value=2
  Constant14 : Constant  Value=350
  Constant15 : Constant  Value=7000
  Constant16 : Constant  Value=1500
  Constant2 : Constant  Value=2048
  Constant3 : Constant  Value=8192
  Constant4 : Constant
  Constant5 : Constant  Value=512
  Constant6 : Constant  Value=256
  Constant7 : Constant  Value=128
  Constant8 : Constant  Value=64
  Constant9 : Constant  Value=32
  Data Type Conversion : DataTypeConversion  OutDataTypeStr=boolean
  Delay : Delay  DelayLength=1  InitialCondition=0
  Detect Change : simulink/Logic and Bit Operations/Detect Change  vinit=0  OutDataTypeStr=boolean
  Ground : Ground
  Integrator : Integrator  ExternalReset=rising
  Integrator1 : Integrator  ExternalReset=rising
  Logical Operator : Logic  Operator=OR  AllPortsSameDT=off  OutDataTypeStr=boolean
  Logical Operator1 : Logic  Operator=NOT  AllPortsSameDT=off  OutDataTypeStr=boolean
  Multiport Switch : MultiPortSwitch  Inputs=4
  Product{,1..12} (13 alike) : Product
  Relational Operator{,1..3,5..13} (13 alike) : RelationalOperator  OutDataTypeStr=boolean  RndMeth=Simplest
  Relational Operator14 : RelationalOperator  Operator=>  OutDataTypeStr=boolean  RndMeth=Simplest
  Relational Operator4 : RelationalOperator  Operator===  OutDataTypeStr=boolean  RndMeth=Simplest
  S-R Flip-Flop : simulink_extras/Flip Flops/S-R Flip-Flop  initial_condition=0
  S-R Flip-Flop1 : simulink_extras/Flip Flops/S-R Flip-Flop  initial_condition=0
  Saturation : Saturate  UpperLimit=10000  LowerLimit=0
  Switch : Switch  Criteria=u2 > Threshold
  Switch1 : Switch  Criteria=u2 > Threshold
  Terminator : Terminator
  Terminator1 : Terminator
  cnst_change : Constant  Value=4758
  mode : Constant
  add_0.1_MW : Outport
  add_0.2_MW : Outport  Port=2
  add_0.4_MW : Outport  Port=3
  add_0.8_MW : Outport  Port=4
  add_1.6_MW : Outport  Port=5
  add_3.2_MW : Outport  Port=6
  add_6.4_MW : Outport  Port=7
  add_12.8_MW : Outport  Port=8
  add_25.6_MW : Outport  Port=9
  add_51.2_MW : Outport  Port=10
  add_102.4_MW : Outport  Port=11
  add_204.8_MW : Outport  Port=12
  add_409.6_MW : Outport  Port=13
  add_819.2_MW : Outport  Port=14
  wires:
  Constant3/1 -> Relational Operator3/2, Product3/2
  Add2/1 -> Relational Operator4/1
  Relational Operator2/1 -> Product2/1, add_409.6_MW/1
  Add1/1 -> Relational Operator1/1, Add/1
  Constant1/1 -> Relational Operator2/2, Product2/2
  Product2/1 -> Add1/2
  Relational Operator4/1 -> add_0.1_MW/1
  Constant4/1 -> Relational Operator4/2
  Product1/1 -> Add/2
  Product/1 -> Add2/2
  Add/1 -> Add4/1, Relational Operator/1
  Relational Operator/1 -> add_102.4_MW/1, Product4/1
  Constant2/1 -> Relational Operator1/2, Product1/2
  Relational Operator1/1 -> Product1/1, add_204.8_MW/1
  Constant/1 -> Product4/2, Relational Operator/2
  Product3/1 -> Add3/2
  Add3/1 -> Relational Operator2/1, Add1/1
  Relational Operator3/1 -> Product3/1, add_819.2_MW/1
  Constant5/1 -> Product5/2, Relational Operator5/2
  Add4/1 -> Add5/1, Relational Operator5/1
  Product4/1 -> Add4/2
  Product5/1 -> Add5/2
  Add5/1 -> Relational Operator6/1, Add6/1
  Constant6/1 -> Product6/2, Relational Operator6/2
  Constant7/1 -> Product7/2, Relational Operator7/2
  Add6/1 -> Add7/1, Relational Operator7/1
  Product6/1 -> Add6/2
  Relational Operator5/1 -> Product5/1, add_51.2_MW/1
  Relational Operator6/1 -> add_25.6_MW/1, Product6/1
  Product7/1 -> Add7/2
  Add7/1 -> Add8/1, Relational Operator8/1
  Constant8/1 -> Product8/2, Relational Operator8/2
  Constant9/1 -> Product9/2, Relational Operator9/2
  Add8/1 -> Add9/1, Relational Operator9/1
  Product8/1 -> Add8/2
  Product9/1 -> Add9/2
  Add9/1 -> Add10/1, Relational Operator10/1
  Constant10/1 -> Product10/2, Relational Operator10/2
  Constant11/1 -> Product11/2, Relational Operator11/2
  Add10/1 -> Add11/1, Relational Operator11/1
  Product10/1 -> Add10/2
  Product11/1 -> Add11/2
  Add11/1 -> Add12/1, Relational Operator12/1
  Constant12/1 -> Product12/2, Relational Operator12/2
  Constant13/1 -> Product/2, Relational Operator13/2
  Add12/1 -> Add2/1, Relational Operator13/1
  Product12/1 -> Add12/2
  Relational Operator7/1 -> add_12.8_MW/1, Product7/1
  Relational Operator8/1 -> add_6.4_MW/1, Product8/1
  Relational Operator9/1 -> add_3.2_MW/1, Product9/1
  Relational Operator10/1 -> add_1.6_MW/1, Product10/1
  Relational Operator11/1 -> add_0.8_MW/1, Product11/1
  Relational Operator12/1 -> add_0.4_MW/1, Product12/1
  Relational Operator13/1 -> add_0.2_MW/1, Product/1
  Constant14/1 -> Integrator/1, Integrator1/1
  Add14/1 -> Switch/1
  Constant15/1 -> Add14/1, Relational Operator14/2
  Relational Operator14/1 -> S-R Flip-Flop/1
  S-R Flip-Flop/1 -> Delay/1, Switch/2
  cnst_change/1 -> Add15/1, Add13/1, Multiport Switch/2
  Integrator/1 -> Add14/2
  mode/1 -> Multiport Switch/1, Detect Change/1
  Saturation/1 -> Add3/1, Relational Operator3/1
  Add13/1 -> Relational Operator14/1, Switch/3, Multiport Switch/3
  Detect Change/1 -> Integrator1/2, S-R Flip-Flop/2, Logical Operator/1
  Logical Operator/1 -> Integrator/2
  Delay/1 -> Logical Operator/2
  Switch/1 -> Multiport Switch/5
  Add15/1 -> Multiport Switch/4
  Integrator1/1 -> Add13/2, Add15/2
  S-R Flip-Flop/2 -> Terminator/1
  Data Type Conversion/1 -> Logical Operator1/1, S-R Flip-Flop1/1
  trip_AOPO2/1 -> Data Type Conversion/1
  S-R Flip-Flop1/1 -> Switch1/2
  Constant16/1 -> Switch1/1
  Switch1/1 -> Add16/2
  Multiport Switch/1 -> Add16/1
  Add16/1 -> Saturation/1
  Logical Operator1/1 -> S-R Flip-Flop1/2
  S-R Flip-Flop1/2 -> Terminator1/1
  Ground/1 -> Switch1/3
